simulink model "forward_converter_myfile"  (R2019a)
settings: Solver=VariableStepAuto  StartTime=0.0  StopTime=0.15  RelTol=1e-3
libraries: powerlib x12
settings Model: Creator=Deepak  LastModifiedBy=Deepak

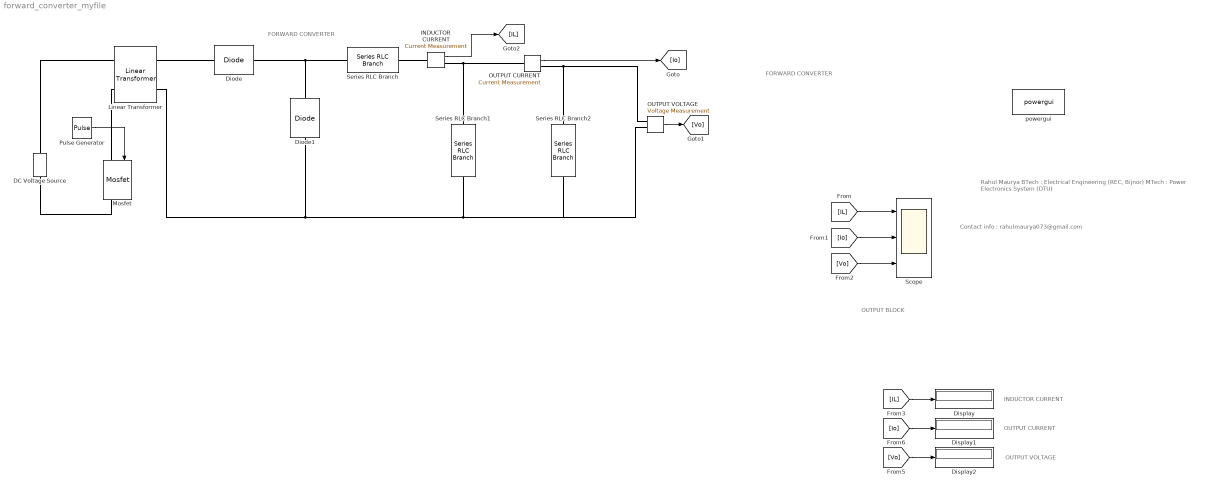
== system forward_converter_myfile ==
  note: OUTPUT VOLTAGE
  note: OUTPUT CURRENT
  note: INDUCTOR CURRENT
  note: FORWARD CONVERTER
  note: OUTPUT BLOCK
  note: Rahul Maurya
      | BTech : Electrical Engineering (REC, Bijnor)
      | MTech : Power Electronics System (DTU)
  note: Contact info : rahulmaurya073@gmail.com
  note: FORWARD CONVERTER
  DC Voltage Source : powerlib/Electrical Sources/DC Voltage Source  Amplitude=300  Measurements=None
      settings: SourceProductName=Simscape Electrical
  Diode : powerlib/Power Electronics/Diode  Ron=0.001  Lon=0  Vf=0  IC=0  UseSnubber=0  Rs=500  Cs=250e-9  Measurements=off
      settings: SourceProductName=Simscape Electrical
  Diode1 : powerlib/Power Electronics/Diode  Ron=0.001  Lon=0  Vf=0  IC=0  UseSnubber=0  Rs=500  Cs=250e-9  Measurements=off
      settings: SourceProductName=Simscape Electrical
  Display : Display
  Display1 : Display
  Display2 : Display
  INDUCTOR CURRENT : powerlib/Measurements/Current Measurement  PhasorSimulation=off  OutputType=Complex  PSBequivalent=0
      settings: SourceProductName=Simscape Electrical
  Linear Transformer : powerlib/Elements/Linear Transformer  UNITS=SI  NominalPower=[ 1000 50e3 ]  winding1=[200 0 0]  winding2=[50 0 0]  ThreeWindings=off  winding3=[3.15e+05 0.7938 0.084225]  RmLm=[inf 96e-3]  Measurements=None  DataType=on
      settings: SourceProductName=Simscape Electrical
  Mosfet : powerlib/Power Electronics/Mosfet  Ron=0.1  Lon=0  Rd=0.01  Vfd=0  IC=0  Rs=1e5  Cs=inf  Measurements=on
      settings: SourceProductName=Simscape Electrical
  OUTPUT CURRENT : powerlib/Measurements/Current Measurement  PhasorSimulation=off  OutputType=Complex  PSBequivalent=0
      settings: SourceProductName=Simscape Electrical
  "OUTPUT VOLTAGE " : powerlib/Measurements/Voltage Measurement  PhasorSimulation=off  OutputType=Complex  PSBequivalent=0
      settings: SourceProductName=Simscape Electrical
  Pulse Generator : DiscretePulseGenerator  PulseType=Time based  Period=1/50e3  PulseWidth=32
  Scope : Scope  NumInputPorts=3
  Series RLC Branch : powerlib/Elements/Series RLC Branch  LConnTagsString=__new0  RConnTagsString=__new0  BranchType=RL  Resistance=0.4  Inductance=3.914e-04  SetiL0=off  InitialCurrent=0  Capacitance=1e-6  Setx0=off  InitialVoltage=0  Measurements=None
      settings: SourceProductName=Simscape Electrical
  Series RLC Branch1 : powerlib/Elements/Series RLC Branch  LConnTagsString=__new0  RConnTagsString=__new0  BranchType=C  Resistance=1  Inductance=1e-3  SetiL0=off  InitialCurrent=0  Capacitance=8.68e-6  Setx0=off  InitialVoltage=0  Measurements=None
      settings: SourceProductName=Simscape Electrical
  Series RLC Branch2 : powerlib/Elements/Series RLC Branch  LConnTagsString=__new0  RConnTagsString=__new0  BranchType=R  Resistance=12  Inductance=1e-3  SetiL0=off  InitialCurrent=0  Capacitance=1e-6  Setx0=off  InitialVoltage=0  Measurements=None
      settings: SourceProductName=Simscape Electrical
  powergui : powerlib/powergui  Priority=1  SimulationMode=Continuous  SampleTime=50e-6  frequency=60  Iterations=50  frequencyindice=0  Pbase=100e6  ErrMax=1e-4  UnitsV=kV  UnitsW=MW  buscounter=0  FunctionMessages=off  echomessages=off  EnableUseOfTLC=off  CurrentSourceSwitches=off  DisableSnubberDevices=off  DisableRonSwitches=off  DisableVfSwitches=off  DisplayEquations=off  AutomaticDiscreteSolvers=off  SolverType=Tustin/Backward Euler (TBE)  Interpol=off  ExternalGateDelay=off  methode=off  Ts=100  x0status=blocks  SPID=on  SwTol=0  HookPort=off  NonlinearTolerance=0  nMaxIteration=15  ContinueOnMaxIteration=off  RestoreLinks=warning  ResistiveCurrentMeasurement=off  Frange=[0:2:500]  Ylog=off  Xlog=on  ShowGrid=off  save=off  variable=ZData  structure=0  ZoomFFT=off  StartTime=0.0  cycles=1  DisplayStyle=1  fundamental=60  FreqAxis=off  MaxFrequency=1000  frequencyindicesteady=1  RmsSteady=1  display=off
      settings: SourceProductName=Simscape Electrical
  wires:
  OUTPUT CURRENT/1 -> [Io]
  "OUTPUT VOLTAGE "/1 -> [Vo]
  INDUCTOR CURRENT/1 -> [IL]
  Pulse Generator/1 -> Mosfet/1
  [IL] -> Scope/1
  [Io] -> Scope/2
  [Vo] -> Scope/3
  [IL] -> Display/1
  [Io] -> Display1/1
  [Vo] -> Display2/1
  connections:
  Linear Transformer/LConn1 -- DC Voltage Source/RConn1
  Mosfet/LConn1 -- Linear Transformer/LConn2
  Mosfet/RConn1 -- DC Voltage Source/LConn1
  Diode/LConn1 -- Linear Transformer/RConn1
  Diode1/RConn1 -- Diode/RConn1 -- Series RLC Branch/LConn1
  INDUCTOR CURRENT/LConn1 -- Series RLC Branch/RConn1
  INDUCTOR CURRENT/RConn1 -- OUTPUT CURRENT/LConn1 -- Series RLC Branch1/LConn1
  Series RLC Branch1/RConn1 -- "OUTPUT VOLTAGE "/LConn2 -- Series RLC Branch2/RConn1 -- Diode1/LConn1 -- Linear Transformer/RConn2
  Series RLC Branch2/LConn1 -- "OUTPUT VOLTAGE "/LConn1 -- OUTPUT CURRENT/RConn1
